simulink model "blank_canvas_118"  (R2025a)
settings: Solver=FixedStepDiscrete  StartTime=0.0  StopTime=2  FixedStep=Ts  RelTol=1e-3
settings Model: Creator=gdudgeon  LastModifiedBy=gdudgeon
settings DataIOCC: SaveOutput=off  SignalLogging=off  DSMLogging=off  SaveTime=off  ReturnWorkspaceOutputs=off
settings RTWCC: GPUComputeCapability=3.5

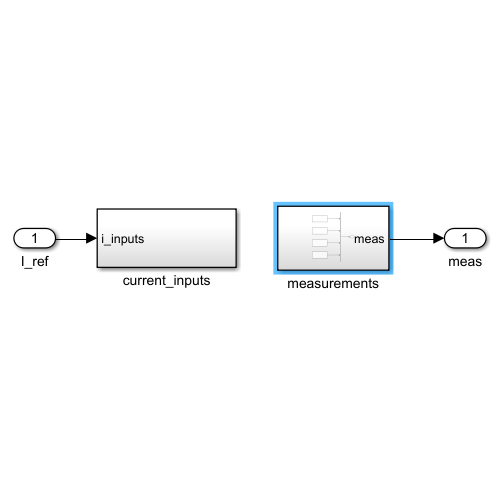
[thumbnail: Simulink's stored preview of the top-level diagram]
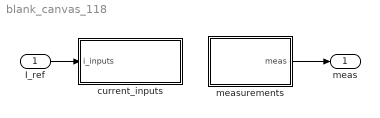
== system blank_canvas_118 ==
  I_ref : Inport
  current_inputs : Subsystem
  measurements : Subsystem
  meas : Outport
  wires:
  measurements/1(meas) -> meas/1
  I_ref/1 -> current_inputs/1(i_inputs)

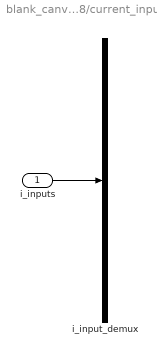
== system blank_canvas_118/current_inputs ==
  i_inputs : Inport
  i_input_demux : Demux  Outputs=2
  wires:
  i_inputs/1 -> i_input_demux/1

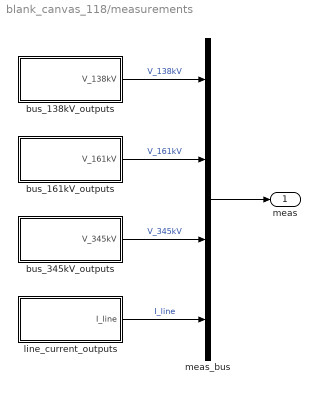
== system blank_canvas_118/measurements ==
  bus_138kV_outputs : Subsystem
  bus_161kV_outputs : Subsystem
  bus_345kV_outputs : Subsystem
  line_current_outputs : Subsystem
  meas_bus : BusCreator  Inputs=4
  meas : Outport
  wires:
  meas_bus/1 -> meas/1
  line_current_outputs/1(I_line) -> meas_bus/4  "I_line"
  bus_345kV_outputs/1(V_345kV) -> meas_bus/3  "V_345kV"
  bus_138kV_outputs/1(V_138kV) -> meas_bus/1  "V_138kV"
  bus_161kV_outputs/1(V_161kV) -> meas_bus/2  "V_161kV"

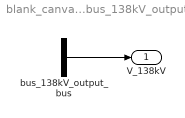
== system blank_canvas_118/measurements/bus_138kV_outputs ==
  bus_138kV_output_bus : BusCreator  Inputs=2
  V_138kV : Outport  VectorParamsAs1DForOutWhenUnconnected=off
  wires:
  bus_138kV_output_bus/1 -> V_138kV/1

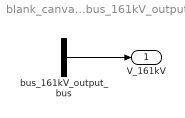
== system blank_canvas_118/measurements/bus_161kV_outputs ==
  bus_161kV_output_bus : BusCreator  Inputs=2
  V_161kV : Outport  VectorParamsAs1DForOutWhenUnconnected=off
  wires:
  bus_161kV_output_bus/1 -> V_161kV/1

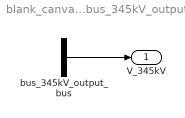
== system blank_canvas_118/measurements/bus_345kV_outputs ==
  bus_345kV_output_bus : BusCreator  Inputs=2
  V_345kV : Outport  VectorParamsAs1DForOutWhenUnconnected=off
  wires:
  bus_345kV_output_bus/1 -> V_345kV/1

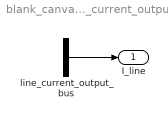
== system blank_canvas_118/measurements/line_current_outputs ==
  line_current_output_bus : BusCreator  Inputs=2
  I_line : Outport  VectorParamsAs1DForOutWhenUnconnected=off
  wires:
  line_current_output_bus/1 -> I_line/1
